simulink model "testing"  (R2022b)
settings: Solver=VariableStepAuto  StartTime=0.0  StopTime=10.0  RelTol=1e-3
libraries: uavalgslib x1
settings Model: SimulationMode=accelerator  Creator=Taim  LastModifiedBy=Taim

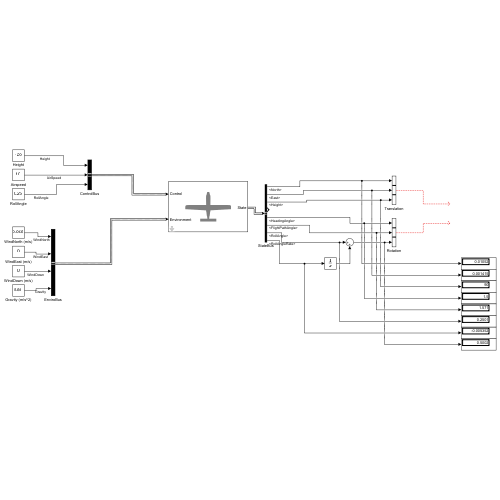
[thumbnail: Simulink's stored preview of the top-level diagram]
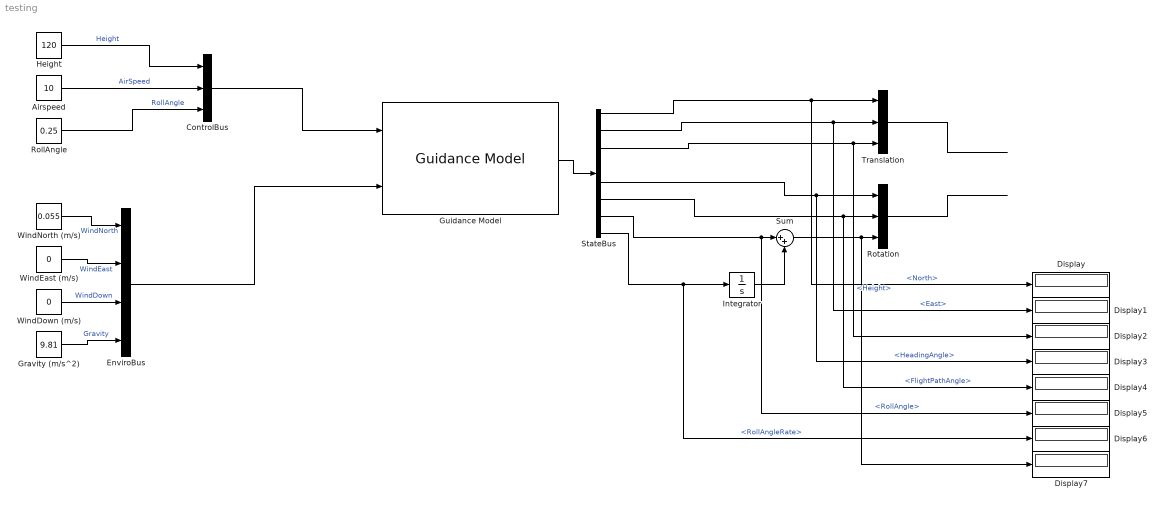
== system testing ==
  Airspeed : Constant  Value=10  OutDataTypeStr=double
  ControlBus : BusCreator  Inputs=3  OutDataTypeStr=Bus: ControlBus  NonVirtualBus=on
  Display{,1..7} (8 alike) : Display
  EnviroBus : BusCreator  Inputs=4  OutDataTypeStr=Bus: EnviroBus  NonVirtualBus=on
  Gravity (m/s^2) : Constant  Value=9.81  OutDataTypeStr=double
  Guidance Model : uavalgslib/Guidance Model  ModelType=FixedWingGuidance  SpecifiedDataType=double  SimulateUsing=Code generation  InitialWorldPositionMultirotor=[0; 0; 0]  InitialWorldVelocityMultirotor=[0; 0; 0]  InitialEulerZYXMultirotor=[0; 0; 0]  InitialBodyAngularRateRPYMultirotor=[0; 0; 0]  InitialThrustMultirotor=0  InitialNorthFixedWing=0  InitialEastFixedWing=0  InitialHeightFixedWing=0  InitialAirSpeedFixedWing=0  InitialHeadingAngleFixedWing=0  InitialFlightPathAngleFixedWing=0  InitialRollAngleFixedWing=0  InitialRollAngleRateFixedWing=0  PDRollMultirotor=[3402.97,116.67]  PDPitchMultirotor=[3402.97, 116.67]  PYawRateMultirotor=1950  PThrustMultirotor=3900  MassMultirotor=0.1  PHeightFixedWing=3.9  PHeadingAngleFixedWing=3.9  PFlightPathAngleFixedWing=39  PDRollFixedWing=[3402.97, 116.67]  PAirSpeedFixedWing=1  FlightPathAngleLimitsFixedWing=[-pi/2, pi/2]  StateBusName='StateBus'  ControlBusName='ControlBus'  EnvironmentBusName='EnviroBus'  DataType=double
  Height : Constant  Value=120  OutDataTypeStr=double
  Integrator : Integrator
  RollAngle : Constant  Value=0.25  OutDataTypeStr=double
  Rotation : Concatenate  NumInputs=3
  StateBus : BusSelector  OutputSignals=North,East,Height,AirSpeed,HeadingAngle,FlightPathAngle,RollAngle,RollAngleRate
  Sum : Sum  Inputs=|++
  Translation : Concatenate  NumInputs=3
  WindDown (m/s) : Constant  Value=0
  WindEast (m/s) : Constant  Value=0
  WindNorth (m/s) : Constant  Value=0.055
  wires:
  Airspeed/1 -> ControlBus/2  "AirSpeed"
  Height/1 -> ControlBus/1  "Height"
  RollAngle/1 -> ControlBus/3  "RollAngle"
  ControlBus/1 -> Guidance Model/1
  Gravity (m/s^2)/1 -> EnviroBus/4  "Gravity"
  WindDown (m/s)/1 -> EnviroBus/3  "WindDown"
  WindEast (m/s)/1 -> EnviroBus/2  "WindEast"
  WindNorth (m/s)/1 -> EnviroBus/1  "WindNorth"
  EnviroBus/1 -> Guidance Model/2
  Guidance Model/1 -> StateBus/1
  StateBus/1 -> Display/1, Translation/1  "<North>"
  StateBus/2 -> Display1/1, Translation/2  "<East>"
  StateBus/3 -> Display2/1, Translation/3  "<Height>"
  StateBus/5 -> Display3/1, Rotation/1  "<HeadingAngle>"
  StateBus/6 -> Display4/1, Rotation/2  "<FlightPathAngle>"
  StateBus/8 -> Display6/1, Integrator/1  "<RollAngleRate>"
  Integrator/1 -> Sum/2
  StateBus/7 -> Display5/1, Sum/1  "<RollAngle>"
  Sum/1 -> Display7/1, Rotation/3
  Translation/1 -> ?
  Rotation/1 -> ?
